simulink model "LowLevel_Arduino"  (R2019b)
settings: Solver=ode3  StartTime=0.0  StopTime=inf  RelTol=1e-3
PreLoadFcn:
  | k_synchronize=2;
InitFcn:
  | k_synchronize=2;
  | lego_drive_closedloop_InitData.mdl = get_param(bdroot,'Name');
  | lego_drive_closedloop_InitData.cs = getActiveConfigSet(lego_drive_closedloop_InitData.mdl);
libraries: arduinolib x11, simulink x2, dspswit3 x2
PreSaveFcn:
  | set_param(gcs, 'Location',[35 56 895 605])
CloseFcn:
  | clear k_synchronize lego_drive_closedloop_InitData
settings Model: SimulationMode=external  ExtModeTrigDuration=2  Creator=The MathWorks, Inc.  LastModifiedBy=SMART PC
settings DataIOCC: LimitDataPoints=on  SaveFormat=Array  ReturnWorkspaceOutputs=off
settings OptimizationCC: ExpressionDepthLimit=2147483647  LifeSpan=Inf  MaxStackSize=64
settings DebuggingCC: UnderspecifiedInitializationDetection=Classic  MergeDetectMultiDrivingBlocksExec=none  InheritedTsInSrcMsg=none  ParameterPrecisionLossMsg=none  FcnCallInpInsideContextMsg=warning  AllowSymbolicDim=off  StateNameClashWarn=warning  SFUnexpectedBacktrackingDiag=warning  SFNoUnconditionalDefaultTransitionDiag=warning  ArithmeticOperatorsInVariantConditions=warning
settings HardwareCC: ProdBitPerInt=16  ProdBitPerPointer=16  ProdBitPerSizeT=16  ProdBitPerPtrDiffT=16  ProdLargestAtomicFloat=None  ProdWordSize=8  ProdHWDeviceType=Atmel->AVR  UseEmbeddedCoderFeatures=off  UseSimulinkCoderFeatures=off
settings ModelReferenceCC: PropagateSignalLabelsOutOfModel=off
settings SFSimCC: SimUseLocalCustomCode=off  CustomCodeUndefinedFunction=UseInterfaceOnly
settings RTWCC: SystemTargetFile=ert.tlc  HardwareBoard=Arduino Mega 2560  TemplateMakefile=ert_default_tmf  RTWVerbose=off  RTWUseLocalCustomCode=off  Toolchain=Arduino AVR v1.6.1  BuildConfiguration=Faster Runs
settings CodeAppCC: StateflowObjectComments=on
settings ERTTargetCC: MultiwordLength=2048  ERTCustomFileBanners=off  SupportContinuousTime=on  SupportNonInlinedSFcns=on  ModelStepFunctionPrototypeControlCompliant=off  ConvertIfToSwitch=off  SuppressUnreachableDefaultCases=off
settings ConfigComp: CovMetricSettings=dw  CovHtmlReporting=on  CovSaveCumulativeToWorkspaceVar=on  CovSaveSingleToWorkspaceVar=on  CovExternalEMLEnable=off  CovSFcnEnable=off

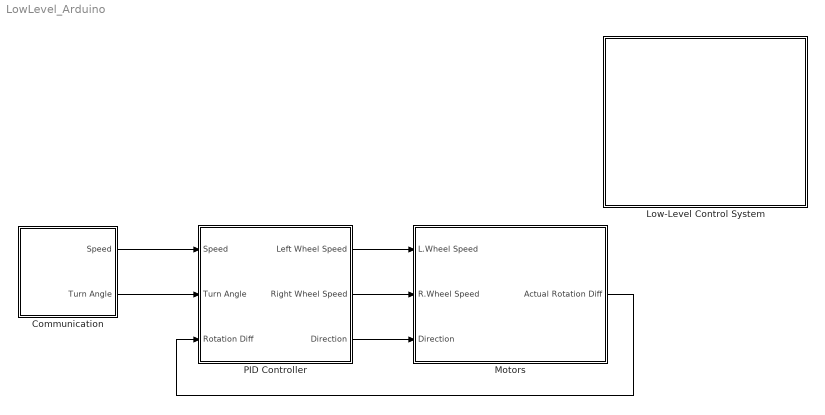
== system LowLevel_Arduino ==
  Communication : Subsystem
  Low-Level Control System : Subsystem
      mask Display: image('icons\arduino_mega.jpg'); % Use "Edit Image" on toolstrip to change.
  Motors : Subsystem  VariantControl=DoSim
      settings: MinAlgLoopOccurrences=on
  PID Controller : Subsystem
  wires:
  Motors/1(Actual Rotation Diff) -> PID Controller/3(Rotation Diff)
  Communication/1(Speed) -> PID Controller/1(Speed)
  Communication/2(Turn Angle) -> PID Controller/2(Turn Angle)
  PID Controller/3(Direction) -> Motors/3(Direction)
  PID Controller/1(Left Wheel Speed) -> Motors/1(L.Wheel Speed)
  PID Controller/2(Right Wheel Speed) -> Motors/2(R.Wheel Speed)

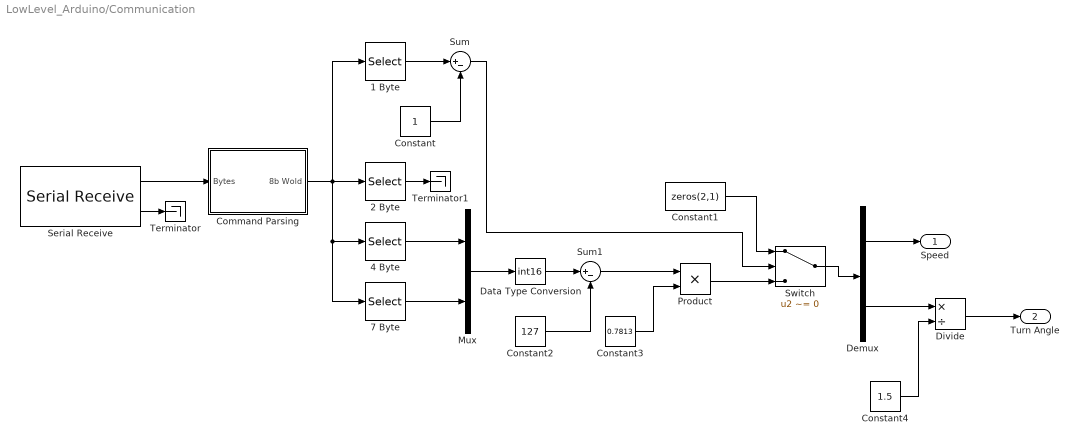
== system LowLevel_Arduino/Communication ==
  1 Byte : Selector  NumberOfDimensions=2  InputPortWidth=3  IndexOptions=Index vector (dialog),Select all  Indices=[1],1  OutputSizes=1,1
  2 Byte : Selector  NumberOfDimensions=2  InputPortWidth=3  IndexOptions=Index vector (dialog),Select all  Indices=[2],1  OutputSizes=1,1
  4 Byte : Selector  NumberOfDimensions=2  InputPortWidth=3  IndexOptions=Index vector (dialog),Select all  Indices=[4],1  OutputSizes=1,1
  7 Byte : Selector  NumberOfDimensions=2  InputPortWidth=3  IndexOptions=Index vector (dialog),Select all  Indices=[7],1  OutputSizes=1,1
  Command Parsing : Subsystem
  Constant : Constant  OutDataTypeStr=uint8
  Constant1 : Constant  Value=zeros(2,1)  OutDataTypeStr=int8
  Constant2 : Constant  Value=127  OutDataTypeStr=uint8
  Constant3 : Constant  Value=0.7813  OutDataTypeStr=double
  Constant4 : Constant  Value=1.5  OutDataTypeStr=double
  Data Type Conversion : DataTypeConversion  OutDataTypeStr=int16
  Demux : Demux  Outputs=2
  Divide : Product  Inputs=*/
  Mux : Mux  Inputs=2
  Product : Product  OutDataTypeStr=int8
  Serial Receive : arduinolib/Serial Receive  portNumber=1  showOutStatus=on  sampleTime=0.001  blockPlatform=arduino
      settings: SourceProductName=Simulink Support Package for Arduino Hardware  SourceProductBaseCode=ARDUINO
  Sum : Sum  Inputs=|+-
  Sum1 : Sum  Inputs=|+-  AccumDataTypeStr=int16
  Switch : Switch  Criteria=u2 ~= 0  OutDataTypeStr=int8
  Terminator : Terminator
  Terminator1 : Terminator
  Speed : Outport
  Turn Angle : Outport  Port=2
  wires:
  Serial Receive/2 -> Terminator/1
  Serial Receive/1 -> Command Parsing/1(Bytes)
  Command Parsing/1(8b Wold) -> 2 Byte/1, 7 Byte/1, 4 Byte/1, 1 Byte/1
  1 Byte/1 -> Sum/1
  Sum/1 -> Switch/2
  Constant/1 -> Sum/2
  Constant1/1 -> Switch/1
  7 Byte/1 -> Mux/2
  2 Byte/1 -> Terminator1/1
  4 Byte/1 -> Mux/1
  Constant2/1 -> Sum1/2
  Sum1/1 -> Product/1
  Constant3/1 -> Product/2
  Data Type Conversion/1 -> Sum1/1
  Demux/1 -> Speed/1
  Switch/1 -> Demux/1
  Mux/1 -> Data Type Conversion/1
  Product/1 -> Switch/3
  Demux/2 -> Divide/1
  Divide/1 -> Turn Angle/1
  Constant4/1 -> Divide/2

== system LowLevel_Arduino/Low-Level Control System ==

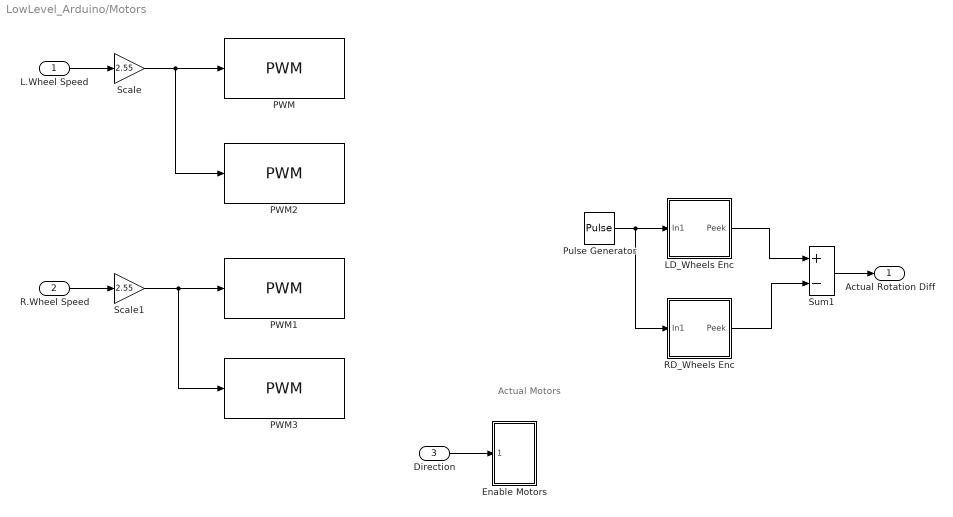
== system LowLevel_Arduino/Motors ==
  note: Actual
      | Motors
  L.Wheel Speed : Inport
  R.Wheel Speed : Inport  Port=2
  Direction : Inport  Port=3
  Enable Motors : Subsystem
  "LD_Wheels Enc " : Subsystem
  PWM : arduinolib/PWM  pinNumber=2  blockPlatform=arduino
  PWM1 : arduinolib/PWM  pinNumber=4  blockPlatform=arduino
  PWM2 : arduinolib/PWM  pinNumber=3  blockPlatform=arduino
  PWM3 : arduinolib/PWM  pinNumber=5  blockPlatform=arduino
  Pulse Generator : DiscretePulseGenerator  PulseType=Time based  Period=0.1  PulseWidth=50
  RD_Wheels Enc : Subsystem
  Scale : Gain  Gain=2.55
  Scale1 : Gain  Gain=2.55
  Sum1 : Sum  Inputs=+-  OutDataTypeStr=Inherit: Same as first input
  Actual Rotation Diff : Outport
  wires:
  R.Wheel Speed/1 -> Scale1/1
  L.Wheel Speed/1 -> Scale/1
  Sum1/1 -> Actual Rotation Diff/1
  Scale/1 -> PWM2/1, PWM/1
  Scale1/1 -> PWM3/1, PWM1/1
  Direction/1 -> Enable Motors/1(Direction)
  "LD_Wheels Enc "/1(Peek) -> Sum1/1
  RD_Wheels Enc/1(Peek) -> Sum1/2
  Pulse Generator/1 -> RD_Wheels Enc/1(In1), "LD_Wheels Enc "/1(In1)

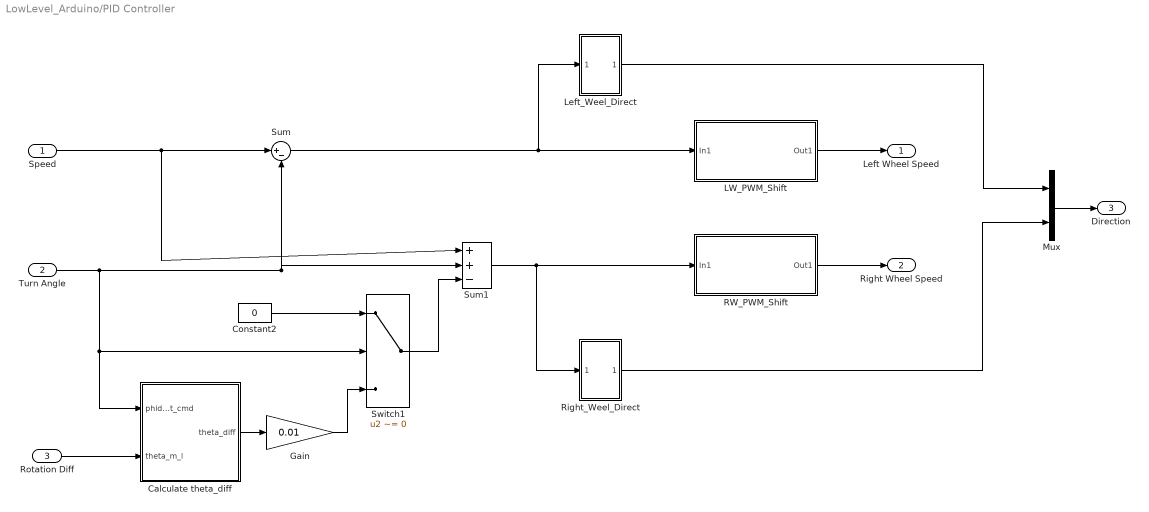
== system LowLevel_Arduino/PID Controller ==
  Speed : Inport
  Turn Angle : Inport  Port=2
  Rotation Diff : Inport  Port=3
  Calculate theta_diff : Subsystem
  Constant2 : Constant  Value=0  OutDataTypeStr=single
  Gain : Gain  Gain=0.01
  LW_PWM_Shift : Subsystem
  Left_Weel_Direct : Subsystem
  Mux : Mux  Inputs=2
  RW_PWM_Shift : Subsystem
  Right_Weel_Direct : Subsystem
  Sum : Sum  Inputs=|+-  OutDataTypeStr=Inherit: Same as first input
  Sum1 : Sum  Inputs=|++-  OutDataTypeStr=Inherit: Same as first input
  Switch1 : Switch  Criteria=u2 ~= 0  OutDataTypeStr=int8
  Left Wheel Speed : Outport
  Right Wheel Speed : Outport  Port=2
  Direction : Outport  Port=3
  wires:
  Constant2/1 -> Switch1/1
  Gain/1 -> Switch1/3
  Speed/1 -> Sum/1, Sum1/1
  Turn Angle/1 -> Sum/2, Sum1/2, Switch1/2, Calculate theta_diff/1(phidot_cmd)
  Rotation Diff/1 -> Calculate theta_diff/2(theta_m_l)
  Calculate theta_diff/1(theta_diff) -> Gain/1
  Sum/1 -> Left_Weel_Direct/1(In1), LW_PWM_Shift/1(In1)
  Sum1/1 -> Right_Weel_Direct/1(In1), RW_PWM_Shift/1(In1)
  Mux/1 -> Direction/1
  Switch1/1 -> Sum1/3
  LW_PWM_Shift/1(Out1) -> Left Wheel Speed/1
  RW_PWM_Shift/1(Out1) -> Right Wheel Speed/1
  Left_Weel_Direct/1(Out1) -> Mux/1
  Right_Weel_Direct/1(Out1) -> Mux/2

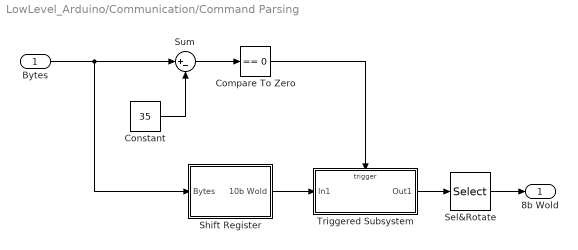
== system LowLevel_Arduino/Communication/Command Parsing ==
  Bytes : Inport
  Compare To Zero : simulink/Logic and Bit Operations/Compare To Zero  relop===  OutDataTypeStr=boolean
  Constant : Constant  Value=35  OutDataTypeStr=uint8
  Sel&Rotate : Selector  NumberOfDimensions=2  InputPortWidth=3  IndexOptions=Index vector (dialog),Select all  Indices=[9:-1:2],1  OutputSizes=1,1
  Shift Register : Subsystem
  Sum : Sum  Inputs=|+-  OutDataTypeStr=int8
  Triggered Subsystem : Subsystem  TreatAsAtomicUnit=on
  8b Wold : Outport
  wires:
  Triggered Subsystem/1(Out1) -> Sel&Rotate/1
  Shift Register/1(10b Wold) -> Triggered Subsystem/1(In1)
  Constant/1 -> Sum/2
  Sum/1 -> Compare To Zero/1
  Compare To Zero/1 -> Triggered Subsystem/Trigger
  Sel&Rotate/1 -> 8b Wold/1
  Bytes/1 -> Sum/1, Shift Register/1(Bytes)

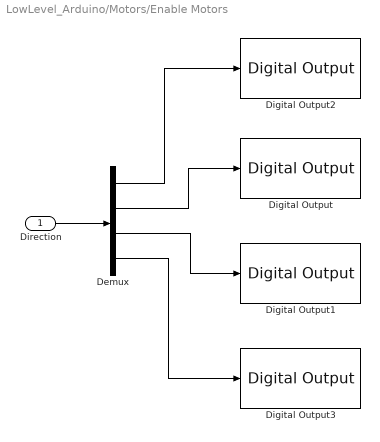
== system LowLevel_Arduino/Motors/Enable Motors ==
  Direction : Inport
  Demux : Demux
  Digital Output : arduinolib/Digital Output  pinNumber=24  blockPlatform=arduino
  Digital Output1 : arduinolib/Digital Output  pinNumber=28  blockPlatform=arduino
  Digital Output2 : arduinolib/Digital Output  pinNumber=22  blockPlatform=arduino
  Digital Output3 : arduinolib/Digital Output  pinNumber=26  blockPlatform=arduino
  wires:
  Demux/2 -> Digital Output/1
  Demux/1 -> Digital Output2/1
  Demux/4 -> Digital Output3/1
  Direction/1 -> Demux/1
  Demux/3 -> Digital Output1/1

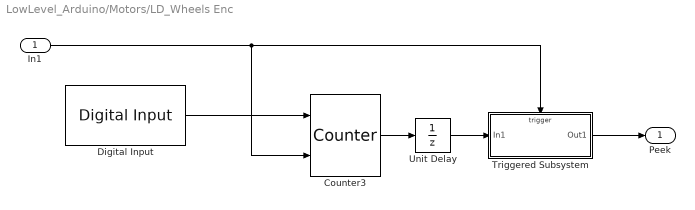
== system LowLevel_Arduino/Motors/LD_Wheels Enc  ==
  In1 : Inport
  Counter3 : dspswit3/Counter  Direction=Up  CountEvent=Rising edge  CounterSize=8 bits  MaxCount=65000  InitialCount=0  Output=Count  HitValue=32  ResetInput=on  SamplesPerFrame=1  Ts=1  CntDtype=uint8  HitDtype=Logical
  Digital Input : arduinolib/Digital Input  pinNumber=11  sampleTime=0.002  blockPlatform=arduino
      settings: SourceProductName=Simulink Support Package for Arduino Hardware
  Triggered Subsystem : Subsystem  TreatAsAtomicUnit=on
  Unit Delay : UnitDelay  SampleTime=-1  HasFrameUpgradeWarning=on
  Peek : Outport
  wires:
  Digital Input/1 -> Counter3/1
  Triggered Subsystem/1(Out1) -> Peek/1
  Counter3/1 -> Unit Delay/1
  In1/1 -> Triggered Subsystem/Trigger, Counter3/2
  Unit Delay/1 -> Triggered Subsystem/1(In1)

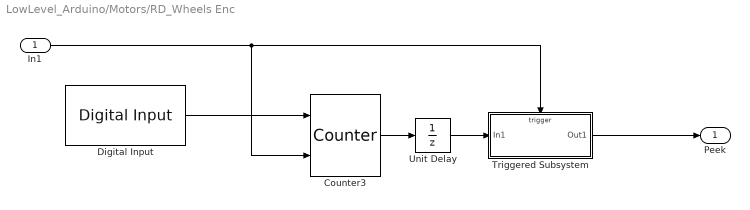
== system LowLevel_Arduino/Motors/RD_Wheels Enc ==
  In1 : Inport
  Counter3 : dspswit3/Counter  Direction=Up  CountEvent=Rising edge  CounterSize=8 bits  MaxCount=65000  InitialCount=0  Output=Count  HitValue=32  ResetInput=on  SamplesPerFrame=1  Ts=1  CntDtype=uint8  HitDtype=Logical
  Digital Input : arduinolib/Digital Input  pinNumber=9  sampleTime=0.002  blockPlatform=arduino
      settings: SourceProductName=Simulink Support Package for Arduino Hardware
  Triggered Subsystem : Subsystem  TreatAsAtomicUnit=on
  Unit Delay : UnitDelay  SampleTime=-1  HasFrameUpgradeWarning=on
  Peek : Outport
  wires:
  Digital Input/1 -> Counter3/1
  Triggered Subsystem/1(Out1) -> Peek/1
  Counter3/1 -> Unit Delay/1
  In1/1 -> Triggered Subsystem/Trigger, Counter3/2
  Unit Delay/1 -> Triggered Subsystem/1(In1)

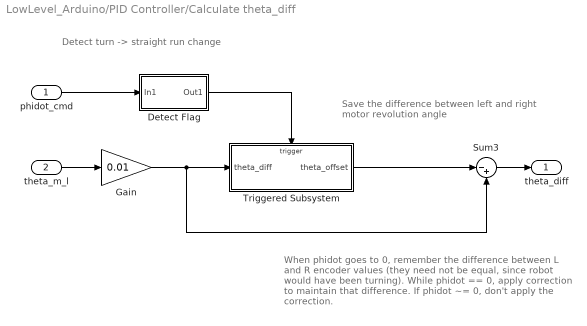
== system LowLevel_Arduino/PID Controller/Calculate theta_diff ==
  note: Detect turn -> straight run change
  note: Save the difference between
      | left and right motor revolution angle
  note: When phidot goes to 0, remember the difference
      | between L and R encoder values (they need not be equal,
      | since robot would have been turning). While phidot == 0,
      | apply correction to maintain that difference.
      | If phidot ~= 0, don't apply the correction.
  phidot_cmd : Inport
  theta_m_l : Inport  Port=2
  Detect Flag : Subsystem
  Gain : Gain  Gain=0.01  ParamDataTypeStr=single
  Sum3 : Sum  Inputs=|-+  OutDataTypeStr=Inherit: Same as first input
  Triggered Subsystem : Subsystem  TreatAsAtomicUnit=on
  theta_diff : Outport
  wires:
  phidot_cmd/1 -> Detect Flag/1(In1)
  theta_m_l/1 -> Gain/1
  Triggered Subsystem/1(theta_offset) -> Sum3/1
  Sum3/1 -> theta_diff/1
  Detect Flag/1(Out1) -> Triggered Subsystem/Trigger
  Gain/1 -> Triggered Subsystem/1(theta_diff), Sum3/2

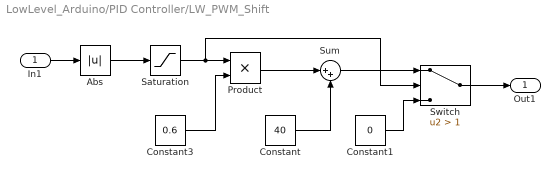
== system LowLevel_Arduino/PID Controller/LW_PWM_Shift ==
  In1 : Inport
  Abs : Abs
  Constant : Constant  Value=40  OutDataTypeStr=uint8
  Constant1 : Constant  Value=0  OutDataTypeStr=uint8
  Constant3 : Constant  Value=0.6
  Product : Product  OutDataTypeStr=uint8
  Saturation : Saturate  UpperLimit=100  LowerLimit=0
      settings: AttributesFormatString=max = %<UpperLimit>\nmin = %<LowerLimit>
  Sum : Sum  Inputs=|++
  Switch : Switch  Criteria=u2 > Threshold  Threshold=1
  Out1 : Outport
  wires:
  Constant3/1 -> Product/2
  In1/1 -> Abs/1
  Product/1 -> Sum/1
  Constant/1 -> Sum/2
  Saturation/1 -> Switch/2, Product/1
  Sum/1 -> Switch/1
  Switch/1 -> Out1/1
  Constant1/1 -> Switch/3
  Abs/1 -> Saturation/1

== system LowLevel_Arduino/PID Controller/Left_Weel_Direct ==
  In1 : Inport
  -->1 : Constant  Value=[0 0]  OutDataTypeStr=boolean
  <--1 : Constant  Value=[1 1]  OutDataTypeStr=boolean
  Switch4 : Switch
  Out1 : Outport
  wires:
  Switch4/1 -> Out1/1
  -->1/1 -> Switch4/1
  <--1/1 -> Switch4/3
  In1/1 -> Switch4/2

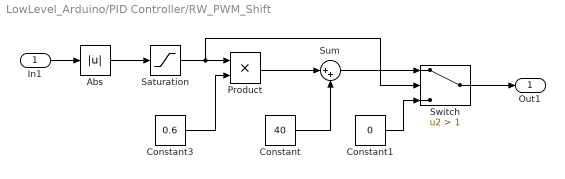
== system LowLevel_Arduino/PID Controller/RW_PWM_Shift ==
  In1 : Inport
  Abs : Abs
  Constant : Constant  Value=40  OutDataTypeStr=uint8
  Constant1 : Constant  Value=0  OutDataTypeStr=uint8
  Constant3 : Constant  Value=0.6
  Product : Product  OutDataTypeStr=uint8
  Saturation : Saturate  UpperLimit=100  LowerLimit=0
      settings: AttributesFormatString=max = %<UpperLimit>\nmin = %<LowerLimit>
  Sum : Sum  Inputs=|++
  Switch : Switch  Criteria=u2 > Threshold  Threshold=1
  Out1 : Outport
  wires:
  Constant3/1 -> Product/2
  Saturation/1 -> Switch/2, Product/1
  In1/1 -> Abs/1
  Product/1 -> Sum/1
  Constant/1 -> Sum/2
  Sum/1 -> Switch/1
  Switch/1 -> Out1/1
  Constant1/1 -> Switch/3
  Abs/1 -> Saturation/1

== system LowLevel_Arduino/PID Controller/Right_Weel_Direct ==
  In1 : Inport
  -->2 : Constant  Value=[1 1]  OutDataTypeStr=boolean
  <--2 : Constant  Value=[0 0]  OutDataTypeStr=boolean
  Switch5 : Switch
  Out1 : Outport
  wires:
  <--2/1 -> Switch5/3
  Switch5/1 -> Out1/1
  -->2/1 -> Switch5/1
  In1/1 -> Switch5/2

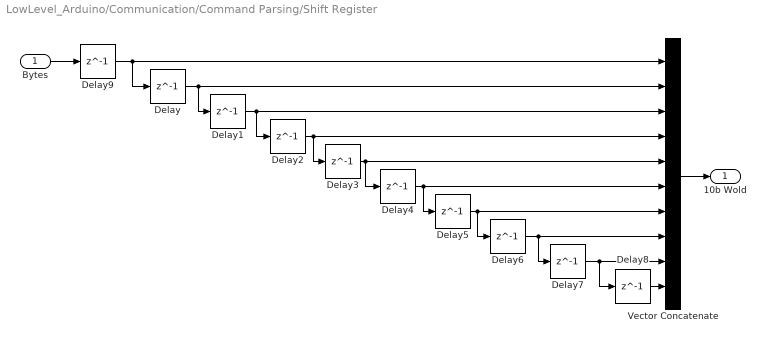
== system LowLevel_Arduino/Communication/Command Parsing/Shift Register ==
  Bytes : Inport
  Delay{,1..9} (10 alike) : Delay  DelayLength=1  InitialCondition=0
  Vector Concatenate : Concatenate  NumInputs=10
  10b Wold : Outport
  wires:
  Vector Concatenate/1 -> 10b Wold/1
  Bytes/1 -> Delay9/1
  Delay/1 -> Delay1/1, Vector Concatenate/2
  Delay1/1 -> Delay2/1, Vector Concatenate/3
  Delay2/1 -> Delay3/1, Vector Concatenate/4
  Delay3/1 -> Delay4/1, Vector Concatenate/5
  Delay4/1 -> Delay5/1, Vector Concatenate/6
  Delay5/1 -> Delay6/1, Vector Concatenate/7
  Delay6/1 -> Delay7/1, Vector Concatenate/8
  Delay7/1 -> Delay8/1, Vector Concatenate/9
  Delay8/1 -> Vector Concatenate/10
  Delay9/1 -> Delay/1, Vector Concatenate/1

== system LowLevel_Arduino/Communication/Command Parsing/Triggered Subsystem ==
  In1 : Inport
  Trigger : TriggerPort  TriggerType=falling  VariantControl=Variant
  Out1 : Outport
  wires:
  In1/1 -> Out1/1

== system LowLevel_Arduino/Motors/LD_Wheels Enc /Triggered Subsystem ==
  In1 : Inport
  Trigger : TriggerPort  VariantControl=Variant
  Out1 : Outport
  wires:
  In1/1 -> Out1/1

== system LowLevel_Arduino/Motors/RD_Wheels Enc/Triggered Subsystem ==
  In1 : Inport
  Trigger : TriggerPort  VariantControl=Variant
  Out1 : Outport
  wires:
  In1/1 -> Out1/1

== system LowLevel_Arduino/PID Controller/Calculate theta_diff/Detect Flag ==
  In1 : Inport
  Compare To Zero : simulink/Logic and Bit Operations/Compare To Zero  relop=~=  OutDataTypeStr=boolean
  Out1 : Outport
  wires:
  In1/1 -> Compare To Zero/1
  Compare To Zero/1 -> Out1/1

== system LowLevel_Arduino/PID Controller/Calculate theta_diff/Triggered Subsystem ==
  theta_diff : Inport  LatchByDelayingOutsideSignal=on
  Trigger : TriggerPort  TriggerType=falling  VariantControl=Variant
  theta_offset : Outport
  wires:
  theta_diff/1 -> theta_offset/1
